simulink model "bp6_model"  (R2019b)
settings: Solver=ode15s  StartTime=0.0  StopTime=2  FixedStep=0.001  RelTol=1e-10  EnableMultiTasking=on
PreLoadFcn:
  | ww=[1e-9 1e7]; N=39; a=-1; b=1;
model workspace (MAT data in the model file):
  a = -0.9999999727
libraries: cstblocks x2
settings Model: Creator=toshiba  LastModifiedBy=xuedi
settings SolverCC: MaxConsecutiveMinStep=100
settings DataIOCC: MaxDataPoints=10000  SaveFormat=Array  SignalLoggingSaveFormat=ModelDataLogs  ReturnWorkspaceOutputs=off
settings OptimizationCC: ExpressionDepthLimit=2147483647  LifeSpan=inf
settings DebuggingCC: UnderspecifiedInitializationDetection=Classic  MergeDetectMultiDrivingBlocksExec=none  FcnCallInpInsideContextMsg=warning  StateNameClashWarn=warning  SFUnexpectedBacktrackingDiag=warning  SFNoUnconditionalDefaultTransitionDiag=warning  SFExecutionAtInitializationDiag=none  ArithmeticOperatorsInVariantConditions=warning
settings HardwareCC: ProdBitPerPointer=32  ProdBitPerSizeT=32  ProdBitPerPtrDiffT=32  ProdLargestAtomicFloat=None  ProdIntDivRoundTo=Undefined  ProdEndianess=Unspecified  ProdWordSize=32  ProdHWDeviceType=32-bit Generic
settings ModelReferenceCC: PropagateSignalLabelsOutOfModel=off
settings SFSimCC: SimUseLocalCustomCode=off  CustomCodeUndefinedFunction=UseInterfaceOnly
settings RTWCC: RTWUseLocalCustomCode=off
settings CodeAppCC: StateflowObjectComments=on
settings GRTTargetCC: TargetLangStandard=C89/C90 (ANSI)  CombineOutputUpdateFcns=off  GRTInterface=on
settings ConfigComp: CovMetricSettings=dw  CovSaveCumulativeToWorkspaceVar=on  CovSaveSingleToWorkspaceVar=on  CovExternalEMLEnable=off

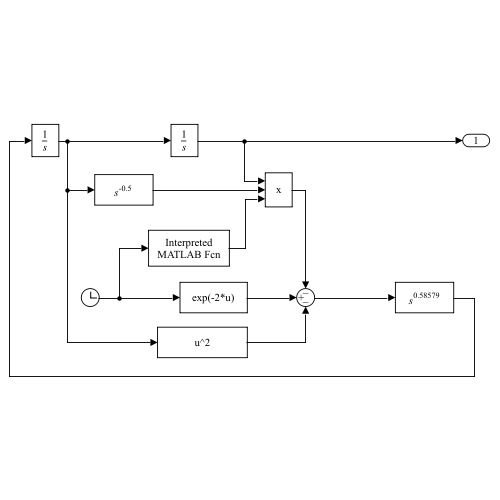
[thumbnail: Simulink's stored preview of the top-level diagram]
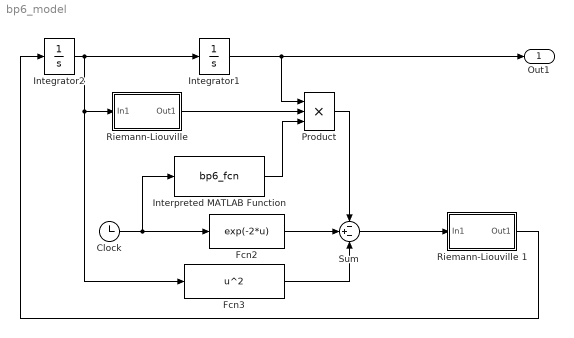
== system bp6_model ==
  Clock : Clock
  Fcn2 : Fcn  Expr=exp(-2*u)
  Fcn3 : Fcn  Expr=u^2
  Integrator1 : Integrator  InitialCondition=b
  Integrator2 : Integrator  InitialCondition=a
  Interpreted MATLAB Function : MATLABFcn  MATLABFcn=bp6_fcn  Output1D=off
  Product : Product  Inputs=***  RndMeth=Zero
  "Riemann-Liouville " : Subsystem  mask{gam=-0.5, ww=ww, n=N, kF1=off, kF=Oustaloup filter}
      mask prompts: gam "Derivative order gamma"; ww "Frequency range [wb,wh]"; n "Apprixmation order"; kF1 "Is a low-pass filter required?"; kF "Filter type"
      mask init:
      | wb=ww(1); wh=ww(2); 
      | if isnumeric(gam), str=['{\its}^{' num2str(gam) '}']; 
      | else, str='{\its}^{\gamma}'; end
      | if kF==1, G=ousta_fod(gam,n,wb,wh);
      | elseif kF==2, G=new_fod(gam,n,wb,wh); 
      | else, G=matsuda_fod(gam,n,wb,wh); end
      | T=1/wh; if kF1==1, G=G*tf(1,[T 1]); end
      mask TypeOptions kF: Oustaloup filter | Modified Oustaloup filter | Matsuda-Fujii filter
      mask Display: disp(str,'texmode','on')
  Riemann-Liouville 1 : Subsystem  mask{gam=2-sqrt(2), ww=ww, n=N, kF1=off, kF=Oustaloup filter}
      mask prompts: gam "Derivative order gamma"; ww "Frequency range [wb,wh]"; n "Apprixmation order"; kF1 "Is a low-pass filter required?"; kF "Filter type"
      mask init: same as bp6_model/Riemann-Liouville 
      mask TypeOptions kF: Oustaloup filter | Modified Oustaloup filter | Matsuda-Fujii filter
      mask Display: disp(str,'texmode','on')
  Sum : Sum  Inputs=-+-
  Out1 : Outport
  wires:
  Integrator1/1 -> Out1/1, Product/1
  Fcn2/1 -> Sum/2
  Sum/1 -> Riemann-Liouville 1/1(In1)
  Integrator2/1 -> Fcn3/1, "Riemann-Liouville "/1(In1), Integrator1/1
  Product/1 -> Sum/1
  Fcn3/1 -> Sum/3
  Clock/1 -> Interpreted MATLAB Function/1, Fcn2/1
  Interpreted MATLAB Function/1 -> Product/3
  "Riemann-Liouville "/1(Out1) -> Product/2
  Riemann-Liouville 1/1(Out1) -> Integrator2/1

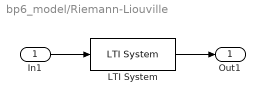
== system bp6_model/Riemann-Liouville  ==
  In1 : Inport
  LTI System : cstblocks/LTI System  sys=G  IC=[]
  Out1 : Outport
  wires:
  LTI System/1 -> Out1/1
  In1/1 -> LTI System/1

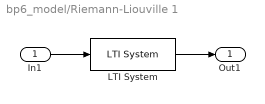
== system bp6_model/Riemann-Liouville 1 ==
  In1 : Inport
  LTI System : cstblocks/LTI System  sys=G  IC=[]
  Out1 : Outport
  wires:
  In1/1 -> LTI System/1
  LTI System/1 -> Out1/1
